simulink model "abs_model"  (R2020b)
settings: Solver=VariableStepAuto  StartTime=0.0  StopTime=15  RelTol=1e-3
InitFcn:
  | g = 32.18;
  | V0 = 88;
  | RR = 15/12
  | kf = 1;
  | M = 50;
  | pbmax = 1500;
  | tb = 0.01;
  | i = 5;
  | slip = (0:.05:1.0);
  | mu = [0 .4 .8 .97 1.0 .98 .96 .94 .92 .9 .88 .855 .83 .81 .79 .77 .75 .73 .72 .71 .7];
  | Control = 1;
undefined symbols (not defined in the file or in its folder): sigbuilder_block
settings Model: Creator=Akshay A H  LastModifiedBy=Akshay A H

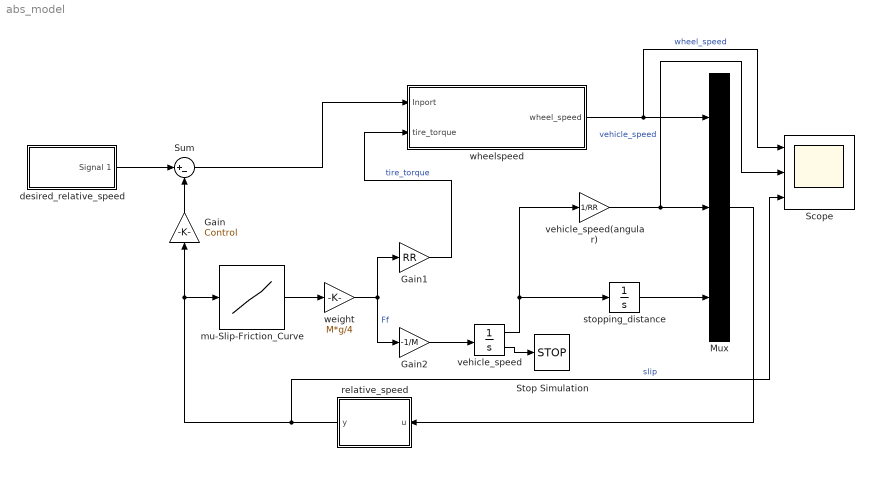
== system abs_model ==
  Gain : Gain  Gain=Control
  Gain1 : Gain  Gain=RR
  Gain2 : Gain  Gain=-1/M
  Mux : Mux  Inputs=3
  Scope : Scope  NumInputPorts=3
  Stop Simulation : Stop
  Sum : Sum  Inputs=|+-
  desired_relative_speed : Subsystem  Tag=STV Subsys  LoadFcn=sigbuilder_block('load');  StartFcn=sigbuilder_block('start');  StopFcn=sigbuilder_block('stop');  ClipboardFcn=sigbuilder_block('clipboard');  mask(Sigbuilder block){tuvar=[0:10]}
      mask help: Simulink:masks:SigbuilderBlock_MD
      mask init:
      | if ~strcmp(get_param(bdroot(gcbh),'SimulationStatus'),'stopped') tuvar = sigbuilder_block('maskInit'); end
      settings: CopyFcn=sigbuilder_block('copy');  DeleteFcn=sigbuilder_block('delete');  ModelCloseFcn=sigbuilder_block('modelClose');  PreSaveFcn=sigbuilder_block('preSave');  PauseFcn=sigbuilder_block('pause');  ContinueFcn=sigbuilder_block('continue');  NameChangeFcn=sigbuilder_block('namechange');  OpenFcn=sigbuilder_block('open',[0 30 960 455.5 ]);  CloseFcn=sigbuilder_block('close');
      mask Display: plot(0, 0, 100, 100,[2, 2, 32, 32, 2], [68, 8, 8, 68, 68],[32, 2], [38, 38], [32, 19, 2],[53, 60, 44], [32, 17, 17, 2],[16, 16, 31, 31]);txt = getActiveGroup(gcbh);text(2, 100, txt,'verticalAlignment', 'top');
  mu-Slip-Friction_Curve : Lookup_n-D  NumberOfTableDimensions=1  BreakpointsForDimension1=slip  Table=mu  SaturateOnIntegerOverflow=on  InputSameDT=on
  relative_speed : MATLAB Function  TreatAsAtomicUnit=on
  stopping_distance : Integrator
  vehicle_speed : Integrator  InitialCondition=V0  LimitOutput=on  UpperSaturationLimit=1000  LowerSaturationLimit=0  ShowSaturationPort=on
  vehicle_speed(angular) : Gain  Gain=1/RR
  weight : Gain  Gain=M*g/4
  wheelspeed : Subsystem
  wires:
  Gain/1 -> Sum/2
  desired_relative_speed/1(Signal 1) -> Sum/1
  mu-Slip-Friction_Curve/1 -> weight/1
  weight/1 -> Gain2/1, Gain1/1  "Ff"
  Gain2/1 -> vehicle_speed/1
  vehicle_speed/2 -> Stop Simulation/1
  Sum/1 -> wheelspeed/1(Inport)
  Gain1/1 -> wheelspeed/2(tire_torque)  "tire_torque"
  wheelspeed/1(wheel_speed) -> Scope/1, Mux/1  "wheel_speed"
  vehicle_speed(angular)/1 -> Scope/2, Mux/2  "vehicle_speed"
  vehicle_speed/1 -> stopping_distance/1, vehicle_speed(angular)/1
  stopping_distance/1 -> Mux/3
  Mux/1 -> relative_speed/1(u)
  relative_speed/1(y) -> Scope/3, mu-Slip-Friction_Curve/1, Gain/1  "slip"

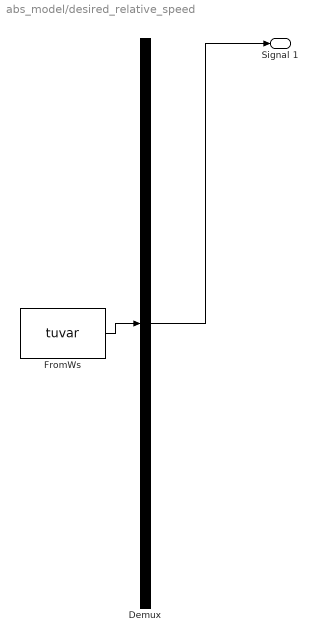
== system abs_model/desired_relative_speed ==
  Demux : Demux  Tag=STV Demux  Outputs=1
      settings: DisplayOption=none
  FromWs : FromWorkspace  Tag=STV FromWs  VariableName=tuvar
      SigBuilderData=|
      | common.afterFinalStr = 'Extrapolate'
      | common.sampleTime = 0
      | dataSet.timeRange = [0 10]
      | dataSet.name = 'Group 1'
      | sbobj.Groups.Name = 'Group 1'
      | sbobj.Groups.Signals.Name = 'Signal 1'
      | sbobj.Groups.Signals.XData = [0 1.99 4 6 6 8.01 8.01 10]
      | sbobj.Groups.Signals.YData = [0.2 0.2 0.2 0.2 0.1999 0.1999 0.2 0.2]
  Signal 1 : Outport  Tag=STV Outport
  wires:
  Demux/1 -> Signal 1/1
  FromWs/1 -> Demux/1

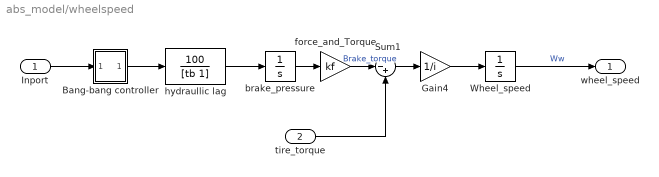
== system abs_model/wheelspeed ==
  Inport : Inport
  tire_torque : Inport  Port=2
  Bang-bang controller : Subsystem  mask(Sign){}
      mask help: y = sign(x)
      mask Help: Sign Function:\n\t\t\ty = 1 if x > 0\n\t\t\ty = 0 if x = 0\n\t\t\ty = -1 if x < 0
      mask Display: plot(-50,-50,50,50,[-50,50],[0,0],[0,0],[-50,50],[-40,0],[-30,-30],[0,40],[30,30])
  Gain4 : Gain  Gain=1/i
  Sum1 : Sum  Inputs=|-+
  Wheel_speed : Integrator  InitialCondition=V0/RR  LimitOutput=on  UpperSaturationLimit=1000  LowerSaturationLimit=0
  brake_pressure : Integrator  LimitOutput=on  UpperSaturationLimit=pbmax  LowerSaturationLimit=0
  force_and_Torque : Gain  Gain=kf
  hydraullic lag : TransferFcn  Numerator=[100]  Denominator=[tb 1]
  wheel_speed : Outport
  wires:
  Bang-bang controller/1(out_1) -> hydraullic lag/1
  Wheel_speed/1 -> wheel_speed/1  "Ww"
  brake_pressure/1 -> force_and_Torque/1
  Inport/1 -> Bang-bang controller/1(in_1)
  hydraullic lag/1 -> brake_pressure/1
  tire_torque/1 -> Sum1/2
  Gain4/1 -> Wheel_speed/1
  force_and_Torque/1 -> Sum1/1  "Brake_torque"
  Sum1/1 -> Gain4/1

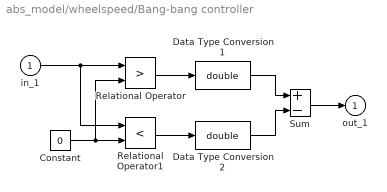
== system abs_model/wheelspeed/Bang-bang controller ==
  in_1 : Inport
  Constant : Constant  Value=0
  Data Type Conversion1 : DataTypeConversion  OutDataTypeStr=double  SaturateOnIntegerOverflow=on  RndMeth=Zero
  Data Type Conversion2 : DataTypeConversion  OutDataTypeStr=double  SaturateOnIntegerOverflow=on  RndMeth=Zero
  Relational Operator : RelationalOperator  Operator=>  OutDataTypeStr=boolean  RndMeth=Nearest  InputSameDT=on
  Relational Operator1 : RelationalOperator  Operator=<  OutDataTypeStr=boolean  RndMeth=Nearest  InputSameDT=on
  Sum : Sum  Inputs=+-  InputSameDT=on  SaturateOnIntegerOverflow=on  OutDataTypeStr=Inherit: Same as first input
  out_1 : Outport  InitialOutput=0  VectorParamsAs1DForOutWhenUnconnected=off
  wires:
  Data Type Conversion2/1 -> Sum/2
  Data Type Conversion1/1 -> Sum/1
  Sum/1 -> out_1/1
  Relational Operator/1 -> Data Type Conversion1/1
  Relational Operator1/1 -> Data Type Conversion2/1
  Constant/1 -> Relational Operator/2, Relational Operator1/2
  in_1/1 -> Relational Operator1/1, Relational Operator/1

== matlab function abs_model/relative_speed ==
  data: u input; y output
function y = fcn(u)
y = 1.0-u(1)/u(2)+(u(2)==0)*eps;
